simulink model "INS"  (R2021a)
settings: configuration reference "ins_config" (kept outside this file)
undefined symbols (not defined in the file): DiscIntNeverNeededParam, INS_CONST, INS_EXPORT, INS_EXPORT_VALUE, INS_PARAM
libraries: simulink x111, FMT_Model_Lib x36
(part 3 of 5)

== system INS/Data_Fusion/Rotation_Filter/RF_Data_PreProcess/Attitude_Reset/Reset Heading ==
  note: When GPS is valid at first time, the mag data will be compensated with WMM data,
      | so we need reset attitude.
  GPS_valid : Inport
  Add : Sum  AccumDataTypeStr=uint32
  Data Type Conversion : DataTypeConversion  OutDataTypeStr=uint32
  Delay : Delay  DelayLength=1
  Detect Rise Positive1 : simulink/Logic and Bit Operations/Detect Rise Positive  vinit=0  OutDataTypeStr=boolean
  Saturation : Saturate  UpperLimit=1  LowerLimit=0
  reset : Outport  VectorParamsAs1DForOutWhenUnconnected=off
  wires:
  Delay/1 -> Add/2
  Data Type Conversion/1 -> Add/1
  GPS_valid/1 -> Data Type Conversion/1
  Detect Rise Positive1/1 -> reset/1
  Add/1 -> Saturation/1
  Saturation/1 -> Detect Rise Positive1/1, Delay/1

== system INS/Data_Fusion/Rotation_Filter/RF_Data_PreProcess/Attitude_Reset/sample_valid ==
  valid : Inport
  Add : Sum  AccumDataTypeStr=uint32
  Data Type Conversion : DataTypeConversion  OutDataTypeStr=uint32
  Delay : Delay  DelayLength=1
  Saturation : Saturate  UpperLimit=10000  LowerLimit=0
  valid_samples : simulink/Logic and Bit Operations/Compare To Constant  relop=>  const=50  OutDataTypeStr=boolean
  sample_valid : Outport  VectorParamsAs1DForOutWhenUnconnected=off
  wires:
  Add/1 -> Saturation/1
  valid_samples/1 -> sample_valid/1
  Delay/1 -> Add/2
  valid/1 -> Data Type Conversion/1
  Data Type Conversion/1 -> Add/1
  Saturation/1 -> valid_samples/1, Delay/1

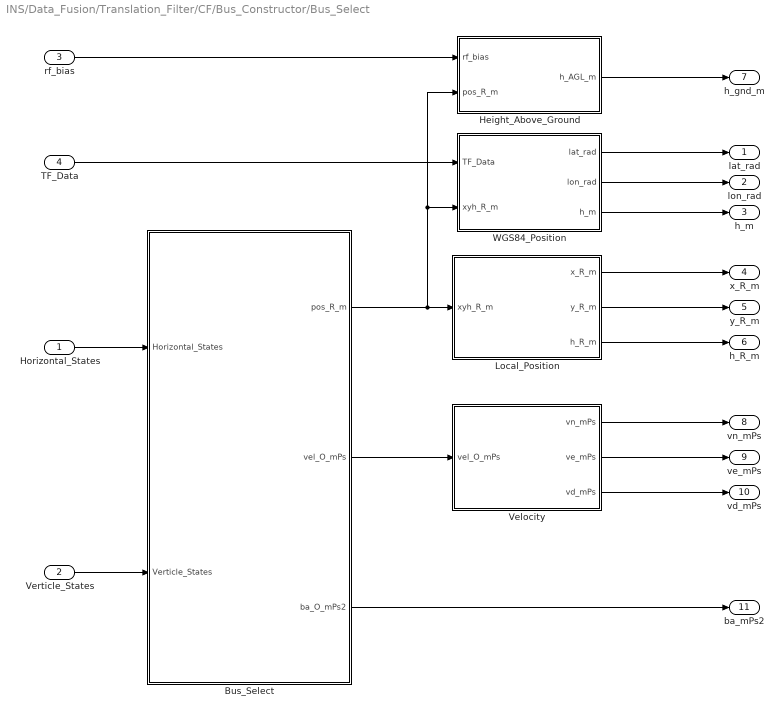
== system INS/Data_Fusion/Translation_Filter/CF/Bus_Constructor/Bus_Select ==
  Horizontal_States : Inport
  Verticle_States : Inport  Port=2
  rf_bias : Inport  Port=3
  TF_Data : Inport  Port=4
  Bus_Select : Subsystem
  Height_Above_Ground : Subsystem
  Local_Position : Subsystem
  Velocity : Subsystem
  WGS84_Position : Subsystem
  lat_rad : Outport  VectorParamsAs1DForOutWhenUnconnected=off
  lon_rad : Outport  Port=2  VectorParamsAs1DForOutWhenUnconnected=off
  h_m : Outport  Port=3  VectorParamsAs1DForOutWhenUnconnected=off
  x_R_m : Outport  Port=4  VectorParamsAs1DForOutWhenUnconnected=off
  y_R_m : Outport  Port=5  VectorParamsAs1DForOutWhenUnconnected=off
  h_R_m : Outport  Port=6  VectorParamsAs1DForOutWhenUnconnected=off
  h_gnd_m : Outport  Port=7  VectorParamsAs1DForOutWhenUnconnected=off
  vn_mPs : Outport  Port=8  VectorParamsAs1DForOutWhenUnconnected=off
  ve_mPs : Outport  Port=9  VectorParamsAs1DForOutWhenUnconnected=off
  vd_mPs : Outport  Port=10  VectorParamsAs1DForOutWhenUnconnected=off
  ba_mPs2 : Outport  Port=11  VectorParamsAs1DForOutWhenUnconnected=off
  wires:
  WGS84_Position/1(lat_rad) -> lat_rad/1
  TF_Data/1 -> WGS84_Position/1(TF_Data)
  WGS84_Position/2(lon_rad) -> lon_rad/1
  WGS84_Position/3(h_m) -> h_m/1
  Local_Position/1(x_R_m) -> x_R_m/1
  Local_Position/2(y_R_m) -> y_R_m/1
  Local_Position/3(h_R_m) -> h_R_m/1
  Bus_Select/1(pos_R_m) -> Local_Position/1(xyh_R_m), Height_Above_Ground/2(pos_R_m), WGS84_Position/2(xyh_R_m)
  Horizontal_States/1 -> Bus_Select/1(Horizontal_States)
  Verticle_States/1 -> Bus_Select/2(Verticle_States)
  Bus_Select/3(ba_O_mPs2) -> ba_mPs2/1
  Height_Above_Ground/1(h_AGL_m) -> h_gnd_m/1
  Bus_Select/2(vel_O_mPs) -> Velocity/1(vel_O_mPs)
  Velocity/1(vn_mPs) -> vn_mPs/1
  Velocity/2(ve_mPs) -> ve_mPs/1
  Velocity/3(vd_mPs) -> vd_mPs/1
  rf_bias/1 -> Height_Above_Ground/1(rf_bias)

== system INS/Data_Fusion/Translation_Filter/CF/Horizontal_Filter/Correct ==
  X_Predict : Inport
  TF_Data : Inport  Port=2
  GPS Correct : Subsystem
  OptFlow Correct : Subsystem
  X_Next : Outport  VectorParamsAs1DForOutWhenUnconnected=off
  wires:
  GPS Correct/1(X_Next) -> X_Next/1
  X_Predict/1 -> OptFlow Correct/1(X_Predict)
  OptFlow Correct/1(X_Next) -> GPS Correct/1(X_Predict)
  TF_Data/1 -> GPS Correct/2(TF_Data), OptFlow Correct/2(TF_Data)

== system INS/Data_Fusion/Translation_Filter/CF/Horizontal_Filter/Predict ==
  X_Prio : Inport
  Rotation_Data : Inport  Port=2
  TF_Data : Inport  Port=3
  Propagate : Subsystem
  Update : Subsystem
  X_Predict : Outport  VectorParamsAs1DForOutWhenUnconnected=off
  wires:
  X_Prio/1 -> Propagate/1(X_prio)
  TF_Data/1 -> Propagate/2(TF_Data)
  Propagate/1(X) -> Update/1(X_Prio)
  Rotation_Data/1 -> Update/2(Rotation_Data)
  Update/1(X_Predict) -> X_Predict/1

== system INS/Data_Fusion/Translation_Filter/CF/Verticle_Filter/Correct ==
  X_Predict : Inport
  TF_Data : Inport  Port=2
  Baro_Correct : Subsystem
  GPS_Correct : Subsystem
  Rf_Correct : Subsystem
  X_Next : Outport  VectorParamsAs1DForOutWhenUnconnected=off
  rf_bias : Outport  Port=2  VectorParamsAs1DForOutWhenUnconnected=off
  wires:
  TF_Data/1 -> Rf_Correct/2(TF_Data), GPS_Correct/2(TF_Data), Baro_Correct/2(TF_Data)
  X_Predict/1 -> Baro_Correct/1(X_Predict)
  Baro_Correct/1(X_Next) -> GPS_Correct/1(X_Predict)
  GPS_Correct/1(X_Next) -> Rf_Correct/1(X_Predict)
  Rf_Correct/1(X_Next) -> X_Next/1
  Rf_Correct/2(rf_bias) -> rf_bias/1

== system INS/Data_Fusion/Translation_Filter/CF/Verticle_Filter/Predict ==
  X_Prio : Inport
  Rotation_Data : Inport  Port=2
  TF_Data : Inport  Port=3
  Propagate : Subsystem
  Update : Subsystem
  X_Predict : Outport  VectorParamsAs1DForOutWhenUnconnected=off
  wires:
  X_Prio/1 -> Propagate/1(X_Prio)
  TF_Data/1 -> Propagate/2(TF_Data)
  Propagate/1(X) -> Update/1(X_Prio)
  Rotation_Data/1 -> Update/2(Rotation_Data)
  Update/1(X_Predict) -> X_Predict/1

== system INS/Data_Fusion/Translation_Filter/TF_Data_PreProcess/Sensor_Process/Sensor_Select ==
  Sensor_Status : Inport
  Bus Creator : BusCreator  Inputs=2
  Horizontal_Sensor_Select : Subsystem
  Vertical_Sensor_Select : Subsystem
  Sensor_Select : Outport  VectorParamsAs1DForOutWhenUnconnected=off
  wires:
  Sensor_Status/1 -> Vertical_Sensor_Select/1(Sensor_Status), Horizontal_Sensor_Select/1(Sensor_Status)
  Bus Creator/1 -> Sensor_Select/1
  Horizontal_Sensor_Select/1(horizon_select) -> Bus Creator/1  "horizon_select"
  Vertical_Sensor_Select/1(vert_select) -> Bus Creator/2  "vert_select"

== system INS/Data_Fusion/Translation_Filter/TF_Data_PreProcess/Sensor_Process/TF_Sensor_Measures ==
  Sensor_Data : Inport
  Rotation_Data : Inport  Port=2
  Barometer_Meas : Subsystem
  Bus Creator : BusCreator  Inputs=4
  GPS_Meas : Subsystem
  OpticalFlow_Meas : Subsystem
  Rangefinder_Meas : Subsystem
  Sensor_Meas : Outport  VectorParamsAs1DForOutWhenUnconnected=off
  wires:
  Bus Creator/1 -> Sensor_Meas/1
  Sensor_Data/1 -> OpticalFlow_Meas/1(Sensor_Data), Rangefinder_Meas/1(Sensor_Data), Barometer_Meas/1(Sensor_Data), GPS_Meas/1(Sensor_Data)
  GPS_Meas/1(GPS_Meas) -> Bus Creator/1  "GPS_Meas"
  Barometer_Meas/1(Baro_Meas) -> Bus Creator/2  "Baro_Meas"
  Rangefinder_Meas/1(Rf_Meas) -> Bus Creator/3  "Rf_Meas"
  OpticalFlow_Meas/1(OptFlow_Meas) -> Bus Creator/4  "OptFlow_Meas"
  Rotation_Data/1 -> OpticalFlow_Meas/2(Rotation_Data)

== system INS/Data_Fusion/Translation_Filter/TF_Data_PreProcess/Sensor_Process/TF_Sensor_Status ==
  Sensor_Data : Inport
  Barometer_Status : Subsystem
  Bus Creator : BusCreator  Inputs=4
  GPS_Status : Subsystem
  OpticalFlow_Status : Subsystem
  Rangefinder_Status : Subsystem
  Sensor_Status : Outport  VectorParamsAs1DForOutWhenUnconnected=off
  wires:
  Bus Creator/1 -> Sensor_Status/1
  Sensor_Data/1 -> OpticalFlow_Status/1(Sensor_Data), Rangefinder_Status/1(Sensor_Data), Barometer_Status/1(Sensor_Data), GPS_Status/1(Sensor_Data)
  GPS_Status/1(GPS_Status) -> Bus Creator/1  "GPS_Status"
  Barometer_Status/1(Baro_Status) -> Bus Creator/2  "Baro_Status"
  Rangefinder_Status/1(Rf_Status) -> Bus Creator/3  "Rf_Status"
  OpticalFlow_Status/1(OptFlow_Status) -> Bus Creator/4  "OptFlow_Status"

== system INS/Data_Fusion/Translation_Filter/TF_Data_PreProcess/Transfer_Filter_Control/Filter_Reset ==
  note: Height_Reset
  note: Position_Reset
  Sensor_Valid : Inport
  Bus Selector : BusSelector  OutputSignals=xy_R_valid
  Bus Selector1 : BusSelector  OutputSignals=h_R_valid
  Detect Rise Positive : simulink/Logic and Bit Operations/Detect Rise Positive  vinit=0  OutDataTypeStr=boolean
  Detect Rise Positive1 : simulink/Logic and Bit Operations/Detect Rise Positive  vinit=0  OutDataTypeStr=boolean
  pos_reset : Outport  VectorParamsAs1DForOutWhenUnconnected=off
  height_reset : Outport  Port=2  VectorParamsAs1DForOutWhenUnconnected=off
  wires:
  Detect Rise Positive/1 -> pos_reset/1
  Detect Rise Positive1/1 -> height_reset/1
  Bus Selector/1 -> Detect Rise Positive/1  "<xy_R_valid>"
  Bus Selector1/1 -> Detect Rise Positive1/1  "<h_R_valid>"
  Sensor_Valid/1 -> Bus Selector1/1, Bus Selector/1

== system INS/Data_Fusion/Translation_Filter/TF_Data_PreProcess/Transfer_Filter_Control/Sensor_Valid ==
  Sensor_Enable : Inport
  Bus Creator : BusCreator  Inputs=5
  Horizon_Sensor_Valid : Subsystem
  Vertical_Sensor_Valid : Subsystem
  Sensor_Valid : Outport  VectorParamsAs1DForOutWhenUnconnected=off
  wires:
  Horizon_Sensor_Valid/1(lon_lat_valid) -> Bus Creator/1  "lon_lat_valid"
  Horizon_Sensor_Valid/2(xy_R_valid) -> Bus Creator/2  "xy_R_valid"
  Vertical_Sensor_Valid/1(altitude_valid) -> Bus Creator/3  "altitude_valid"
  Vertical_Sensor_Valid/2(h_R_valid) -> Bus Creator/4  "h_R_valid"
  Bus Creator/1 -> Sensor_Valid/1
  Sensor_Enable/1 -> Horizon_Sensor_Valid/1(Sensor_Enable), Vertical_Sensor_Valid/1(Sensor_Enable)
  Vertical_Sensor_Valid/3(h_AGL_valid) -> Bus Creator/5  "h_AGL_valid"

== system INS/Data_Fusion/Translation_Filter/TF_Data_PreProcess/Transfer_Filter_Control/WGS84_Reference ==
  Sensor_Valid : Inport
  Translation_Data : Inport  Port=2
  Sensor_Meas : Inport  Port=3
  Bus_Constructor : Subsystem
  Bus_Select : Subsystem
  Height_Ref : Subsystem
  Position_Ref : Subsystem
  WGS84_Ref : Outport  VectorParamsAs1DForOutWhenUnconnected=off
  wires:
  Bus_Select/2(WGS84_position) -> Position_Ref/4(WGS84_position), Height_Ref/4(WGS84_position)
  Translation_Data/1 -> Height_Ref/1(Translation_Data), Position_Ref/1(Translation_Data)
  Sensor_Valid/1 -> Height_Ref/2(Sensor_Valid), Position_Ref/2(Sensor_Valid)
  Bus_Select/1(WGS84_derivatives) -> Height_Ref/3(WGS84_derivatives), Position_Ref/3(WGS84_derivatives)
  Position_Ref/1(WGS84_pos_ref) -> Bus_Constructor/1(WGS84_pos_ref)
  Position_Ref/2(WGS84_dpos_ref) -> Bus_Constructor/2(WGS84_dpos_ref)
  Height_Ref/1(WGS84_hgt_ref) -> Bus_Constructor/3(WGS84_hgt_ref)
  Height_Ref/2(WGS84_dhgt_ref) -> Bus_Constructor/4(WGS84_dhgt_ref)
  Bus_Constructor/1(WGS84_Ref) -> WGS84_Ref/1
  Sensor_Meas/1 -> Bus_Select/1(Sensor_Meas)

== system INS/Sensor_PreProcess/GPS_PreProcess/Status_Quality/GPS_Status/Ready ==
  valid : Inport
  Saturation : Saturate  UpperLimit=1e4  LowerLimit=0
  Sum : Sum  Inputs=|++  OutDataTypeStr=int32
  Unit Delay : UnitDelay  SampleTime=-1  HasFrameUpgradeWarning=on
  valid_samples : simulink/Logic and Bit Operations/Compare To Constant  relop=>=  const=1000  OutDataTypeStr=boolean
  ready : Outport  VectorParamsAs1DForOutWhenUnconnected=off
  wires:
  valid_samples/1 -> ready/1
  Sum/1 -> Saturation/1
  Unit Delay/1 -> valid_samples/1, Sum/2
  Saturation/1 -> Unit Delay/1
  valid/1 -> Sum/1

== system INS/Sensor_PreProcess/MAG_PreProcess/Mag_Data_Process/Mag_Quality_Estimate/Mag_Quality ==
  nominal_inc_deg : Inport
  mag_normalized_O : Inport  Port=2
  Inclination_Quality_Estimate : Subsystem
  Intensity_Quality_Estimate : Subsystem
  MinMax : MinMax  Inputs=2
  Second Order LPF : FMT_Model_Lib/Filter/Second Order LPF  fc=5  zeta=0.707
      settings: SourceProductName=FMT Toolbox
  mag_quality : Outport  VectorParamsAs1DForOutWhenUnconnected=off
  wires:
  Intensity_Quality_Estimate/1(intensity_quality) -> MinMax/2  "mag_int_quality"
  nominal_inc_deg/1 -> Inclination_Quality_Estimate/1(nominal_inc_deg)
  Inclination_Quality_Estimate/1(inclination_quality) -> MinMax/1  "mag_inc_quality"
  mag_normalized_O/1 -> Inclination_Quality_Estimate/2(mag_normalized_O), Intensity_Quality_Estimate/1(mag_normalized_O)
  MinMax/1 -> Second Order LPF/1
  Second Order LPF/1 -> mag_quality/1

== system INS/Sensor_PreProcess/MAG_PreProcess/Mag_Data_Process/WMM_Compensation/safe_divide ==
  u1 : Inport
  u2 : Inport  Port=2
  Constant1 : Constant  VectorParams1D=off  OutDataTypeStr=single
  Divide1 : Product  Inputs=*/
  MinMax : MinMax  Function=max  Inputs=2
  y : Outport  VectorParamsAs1DForOutWhenUnconnected=off
  wires:
  MinMax/1 -> Divide1/2
  Constant1/1 -> MinMax/1
  Divide1/1 -> y/1
  u2/1 -> MinMax/2
  u1/1 -> Divide1/1

== system INS/Data_Fusion/Rotation_Filter/AHRS/Correct/Attitude_Correction/Attitude_Correct ==
  Rotation_Data : Inport
  Sensor_Data : Inport  Port=2
  Acc_Correct : Subsystem
  Acc_Estimator : Subsystem
  att_corr_O : Outport  VectorParamsAs1DForOutWhenUnconnected=off
  wires:
  Acc_Estimator/3(acc_est_O_mPs2) -> Acc_Correct/3(acc_est_O_mPs2)  "acc_est_O_mPs2"
  Sensor_Data/1 -> Acc_Estimator/1(Sensor_Data)
  Rotation_Data/1 -> Acc_Estimator/2(Rotation_Data)
  Acc_Correct/1(att_correct) -> att_corr_O/1
  Acc_Estimator/1(acc_meas_valid) -> Acc_Correct/1(acc_meas_valid)  "acc_meas_valid"
  Acc_Estimator/2(acc_meas_O_mPs2) -> Acc_Correct/2(acc_meas_O_mPs2)  "acc_meas_O_mPs2"

== system INS/Data_Fusion/Rotation_Filter/AHRS/Correct/Attitude_Correction/Mag_Correct ==
  Rotation_Data : Inport
  Sensor_Data : Inport  Port=2
  standstill : Inport  Port=3
  Bus Selector1 : BusSelector  OutputSignals=Mag_Data.mag_norm_B,Mag_Data.mag_quality
  Bus Selector4 : BusSelector  OutputSignals=M_OB
  Constant : Constant  Value=INS_PARAM.MAG_AIR_EN
  Logical Operator : Logic  AllPortsSameDT=off  OutDataTypeStr=boolean
  Logical Operator1 : Logic  Operator=OR  AllPortsSameDT=off  OutDataTypeStr=boolean
  MX Product3 : Product  Inputs=3  RndMeth=Simplest
  MX Product4 : Product  Multiplication=Matrix(*)  RndMeth=Simplest
  Relay1 : Relay  OnSwitchValue=0.3  OffSwitchValue=0.2
  Selector4 : Selector  NumberOfDimensions=2  InputPortWidth=3  IndexOptions=Index vector (dialog),Index vector (dialog)  Indices=[2],[1 2 3]  OutputSizes=1,1
  Subsystem : Subsystem  Commented=on
  Z axis : Constant  Value=[0 0 1]  OutDataTypeStr=single
  mag_correct_gain : Gain  Gain=-INS_PARAM.MAG_GAIN  OutDataTypeStr=Inherit: Same as input
  mag_corr_O : Outport  VectorParamsAs1DForOutWhenUnconnected=off
  wires:
  Bus Selector4/1 -> Subsystem/1(M_OB), Selector4/1  "<M_OB>"
  Rotation_Data/1 -> Subsystem/3(Rotation_Data), Bus Selector4/1
  Bus Selector1/2 -> Relay1/1  "<mag_quality>"
  Sensor_Data/1 -> Bus Selector1/1
  mag_correct_gain/1 -> MX Product3/2
  MX Product4/1 -> mag_correct_gain/1  "my_O"
  Selector4/1 -> MX Product4/1
  Relay1/1 -> Logical Operator/1  "mag_enable"
  Logical Operator/1 -> MX Product3/3
  Logical Operator1/1 -> Logical Operator/2
  Constant/1 -> Logical Operator1/1
  standstill/1 -> Logical Operator1/2
  MX Product3/1 -> mag_corr_O/1
  Bus Selector1/1 -> Subsystem/2(mag_B), MX Product4/2  "<mag_norm_B>"
  Z axis/1 -> MX Product3/1

== system INS/Data_Fusion/Translation_Filter/CF/Bus_Constructor/Bus_Select/Bus_Select ==
  Horizontal_States : Inport
  Verticle_States : Inport  Port=2
  Mux : Mux  Inputs=2
  Mux1 : Mux  Inputs=2
  Mux2 : Mux  Inputs=2
  Selector : Selector  InputPortWidth=6  IndexOptions=Index vector (dialog)  Indices=[1 2]  OutputSizes=1
  Selector1 : Selector  InputPortWidth=3  IndexOptions=Index vector (dialog)  Indices=[1]  OutputSizes=1
  Selector2 : Selector  InputPortWidth=6  IndexOptions=Index vector (dialog)  Indices=[3 4]  OutputSizes=1
  Selector3 : Selector  InputPortWidth=3  IndexOptions=Index vector (dialog)  Indices=[2]  OutputSizes=1
  Selector4 : Selector  InputPortWidth=6  IndexOptions=Index vector (dialog)  Indices=[5 6]  OutputSizes=1
  Selector5 : Selector  InputPortWidth=3  IndexOptions=Index vector (dialog)  Indices=[3]  OutputSizes=1
  pos_R_m : Outport  VectorParamsAs1DForOutWhenUnconnected=off
  vel_O_mPs : Outport  Port=2  VectorParamsAs1DForOutWhenUnconnected=off
  ba_O_mPs2 : Outport  Port=3  VectorParamsAs1DForOutWhenUnconnected=off
  wires:
  Selector5/1 -> Mux2/2
  Horizontal_States/1 -> Selector4/1, Selector2/1, Selector/1
  Selector4/1 -> Mux2/1
  Selector2/1 -> Mux1/1
  Selector1/1 -> Mux/2
  Selector/1 -> Mux/1
  Selector3/1 -> Mux1/2
  Mux1/1 -> vel_O_mPs/1
  Verticle_States/1 -> Selector5/1, Selector3/1, Selector1/1
  Mux/1 -> pos_R_m/1
  Mux2/1 -> ba_O_mPs2/1

== system INS/Data_Fusion/Translation_Filter/CF/Bus_Constructor/Bus_Select/Height_Above_Ground ==
  rf_bias : Inport
  pos_R_m : Inport  Port=2
  Selector : Selector  InputPortWidth=3  IndexOptions=Index vector (dialog)  Indices=3  OutputSizes=1
  Sum : Sum  Inputs=|-+
  h_AGL_m : Outport  VectorParamsAs1DForOutWhenUnconnected=off
  wires:
  rf_bias/1 -> Sum/1
  pos_R_m/1 -> Selector/1
  Sum/1 -> h_AGL_m/1
  Selector/1 -> Sum/2

== system INS/Data_Fusion/Translation_Filter/CF/Bus_Constructor/Bus_Select/Local_Position ==
  xyh_R_m : Inport
  Demux : Demux  Outputs=3
  x_R_m : Outport  VectorParamsAs1DForOutWhenUnconnected=off
  y_R_m : Outport  Port=2  VectorParamsAs1DForOutWhenUnconnected=off
  h_R_m : Outport  Port=3  VectorParamsAs1DForOutWhenUnconnected=off
  wires:
  Demux/2 -> y_R_m/1
  Demux/1 -> x_R_m/1
  Demux/3 -> h_R_m/1
  xyh_R_m/1 -> Demux/1

== system INS/Data_Fusion/Translation_Filter/CF/Bus_Constructor/Bus_Select/Velocity ==
  vel_O_mPs : Inport
  Demux : Demux  Outputs=3
  vn_mPs : Outport  VectorParamsAs1DForOutWhenUnconnected=off
  ve_mPs : Outport  Port=2  VectorParamsAs1DForOutWhenUnconnected=off
  vd_mPs : Outport  Port=3  VectorParamsAs1DForOutWhenUnconnected=off
  wires:
  Demux/3 -> vd_mPs/1
  Demux/1 -> vn_mPs/1
  Demux/2 -> ve_mPs/1
  vel_O_mPs/1 -> Demux/1

== system INS/Data_Fusion/Translation_Filter/CF/Bus_Constructor/Bus_Select/WGS84_Position ==
  TF_Data : Inport
  xyh_R_m : Inport  Port=2
  Bus Selector2 : BusSelector  OutputSignals=Sensor_Status.GPS_Status.gps_vaid
  Data Type Conversion2 : DataTypeConversion  OutDataTypeStr=double
  Demux2 : Demux  Outputs=3
  Multiply : Product
  WGS84_Position : Subsystem
  lat_rad : Outport  VectorParamsAs1DForOutWhenUnconnected=off
  lon_rad : Outport  Port=2  VectorParamsAs1DForOutWhenUnconnected=off
  h_m : Outport  Port=3  VectorParamsAs1DForOutWhenUnconnected=off
  wires:
  WGS84_Position/1(WGS84_pos) -> Multiply/2
  TF_Data/1 -> Bus Selector2/1, WGS84_Position/2(TF_Data)
  Bus Selector2/1 -> Data Type Conversion2/1  "<gps_vaid>"
  Data Type Conversion2/1 -> Multiply/1
  Multiply/1 -> Demux2/1
  xyh_R_m/1 -> WGS84_Position/1(xyh_R_m)
  Demux2/1 -> lat_rad/1  "lat_rad"
  Demux2/2 -> lon_rad/1  "lon_rad"
  Demux2/3 -> h_m/1  "h_m"

== system INS/Data_Fusion/Translation_Filter/CF/Horizontal_Filter/Correct/GPS Correct ==
  X_Predict : Inport
  TF_Data : Inport  Port=2
  Bus Selector : BusSelector  OutputSignals=Sensor_Enable.horizon_select.gps_enable
  GPS_Correct : Subsystem
  Switch : Switch  Criteria=u2 > Threshold
  X_Next : Outport  VectorParamsAs1DForOutWhenUnconnected=off
  wires:
  GPS_Correct/1(X_Next) -> Switch/1
  Switch/1 -> X_Next/1
  X_Predict/1 -> GPS_Correct/2(X_Predict), Switch/3
  Bus Selector/1 -> GPS_Correct/Enable, Switch/2  "<gps_enable>"
  TF_Data/1 -> GPS_Correct/1(TF_Data), Bus Selector/1

== system INS/Data_Fusion/Translation_Filter/CF/Horizontal_Filter/Correct/OptFlow Correct ==
  X_Predict : Inport
  TF_Data : Inport  Port=2
  Bus Selector : BusSelector  OutputSignals=Sensor_Enable.horizon_select.optflow_enable
  OptFlow_Correct : Subsystem
  Switch : Switch  Criteria=u2 > Threshold
  X_Next : Outport  VectorParamsAs1DForOutWhenUnconnected=off
  wires:
  OptFlow_Correct/1(X_Next) -> Switch/1
  Switch/1 -> X_Next/1
  X_Predict/1 -> OptFlow_Correct/2(X_Predict), Switch/3
  Bus Selector/1 -> OptFlow_Correct/Enable, Switch/2  "<optflow_enable>"
  TF_Data/1 -> OptFlow_Correct/1(TF_Data), Bus Selector/1

== system INS/Data_Fusion/Translation_Filter/CF/Horizontal_Filter/Predict/Propagate ==
  X_prio : Inport
  TF_Data : Inport  Port=2
  Bus Selector : BusSelector  OutputSignals=TF_Control.pos_reset
  Delay : Delay  DelayLength=1
  States_Init : Subsystem
  Switch : Switch  Criteria=u2 > Threshold
  X : Outport  VectorParamsAs1DForOutWhenUnconnected=off
  wires:
  Delay/1 -> Switch/3
  States_Init/1(X_0) -> Switch/1
  Switch/1 -> X/1
  Bus Selector/1 -> Switch/2  "<pos_reset>"
  TF_Data/1 -> Bus Selector/1, States_Init/1(TF_Data)
  X_prio/1 -> Delay/1

== system INS/Data_Fusion/Translation_Filter/CF/Horizontal_Filter/Predict/Update ==
  X_Prio : Inport
  Rotation_Data : Inport  Port=2
  Add : Sum  Inputs=-+
  Bus Selector2 : BusSelector  OutputSignals=M_OB,acc_B_mPs2
  Constant : Constant  Value=[0;0]  OutDataTypeStr=single
  Gain : Gain  Gain=INS_CONST.dt  OutDataTypeStr=Inherit: Same as input
  Multiply : Product  Multiplication=Matrix(*)
  Mux : Mux  Inputs=3
  Reshape : Reshape  OutputDimensionality=Customize  OutputDimensions=[6,1]
  Selector : Selector  InputPortWidth=3  IndexOptions=Index vector (dialog)  Indices=[1 2]  OutputSizes=1
  Selector1 : Selector  InputPortWidth=6  IndexOptions=Index vector (dialog)  Indices=[3 4]  OutputSizes=1
  Selector2 : Selector  InputPortWidth=6  IndexOptions=Index vector (dialog)  Indices=[5 6]  OutputSizes=1
  Sum : Sum  Inputs=++|
  X_Predict : Outport  VectorParamsAs1DForOutWhenUnconnected=off
  wires:
  Rotation_Data/1 -> Bus Selector2/1
  Bus Selector2/1 -> Multiply/1  "<M_OB>"
  Multiply/1 -> Selector/1  "acc_O"
  Bus Selector2/2 -> Multiply/2  "<acc_B_mPs2>"
  X_Prio/1 -> Selector1/1, Sum/1, Selector2/1
  Selector/1 -> Add/2
  Selector1/1 -> Mux/1
  Constant/1 -> Mux/3
  Mux/1 -> Reshape/1
  Reshape/1 -> Gain/1
  Sum/1 -> X_Predict/1
  Gain/1 -> Sum/2
  Add/1 -> Mux/2
  Selector2/1 -> Add/1

== system INS/Data_Fusion/Translation_Filter/CF/Verticle_Filter/Correct/Baro_Correct ==
  X_Predict : Inport
  TF_Data : Inport  Port=2
  Baro_Correct : Subsystem
  Bus Selector : BusSelector  OutputSignals=Sensor_Enable.vert_select.baro_enable
  Switch : Switch  Criteria=u2 > Threshold
  X_Next : Outport  VectorParamsAs1DForOutWhenUnconnected=off
  wires:
  Switch/1 -> X_Next/1
  Bus Selector/1 -> Baro_Correct/Enable, Switch/2  "<baro_enable>"
  TF_Data/1 -> Baro_Correct/1(TF_Data), Bus Selector/1
  Baro_Correct/1(X_Next) -> Switch/1
  X_Predict/1 -> Baro_Correct/2(X_Predict), Switch/3

== system INS/Data_Fusion/Translation_Filter/CF/Verticle_Filter/Correct/GPS_Correct ==
  X_Predict : Inport
  TF_Data : Inport  Port=2
  Bus Selector : BusSelector  OutputSignals=Sensor_Enable.vert_select.gps_enable
  GPS_Correct : Subsystem
  Switch : Switch  Criteria=u2 > Threshold
  X_Next : Outport  VectorParamsAs1DForOutWhenUnconnected=off
  wires:
  Switch/1 -> X_Next/1
  Bus Selector/1 -> GPS_Correct/Enable, Switch/2  "<gps_enable>"
  TF_Data/1 -> GPS_Correct/1(TF_Data), Bus Selector/1
  GPS_Correct/1(X_Next) -> Switch/1
  X_Predict/1 -> GPS_Correct/2(X_Predict), Switch/3

== system INS/Data_Fusion/Translation_Filter/CF/Verticle_Filter/Correct/Rf_Correct ==
  X_Predict : Inport
  TF_Data : Inport  Port=2
  Bus Selector : BusSelector  OutputSignals=Sensor_Enable.vert_select.rf_enable
  Rangefinder_Correct : Subsystem
  Switch : Switch  Criteria=u2 > Threshold
  X_Next : Outport  VectorParamsAs1DForOutWhenUnconnected=off
  rf_bias : Outport  Port=2  VectorParamsAs1DForOutWhenUnconnected=off
  wires:
  Switch/1 -> X_Next/1
  Bus Selector/1 -> Rangefinder_Correct/Enable, Switch/2  "<rf_enable>"
  TF_Data/1 -> Rangefinder_Correct/1(TF_Data), Bus Selector/1
  Rangefinder_Correct/1(X_Next) -> Switch/1
  X_Predict/1 -> Rangefinder_Correct/2(X_Predict), Switch/3
  Rangefinder_Correct/2(rf_bias) -> rf_bias/1

== system INS/Data_Fusion/Translation_Filter/CF/Verticle_Filter/Predict/Propagate ==
  X_Prio : Inport
  TF_Data : Inport  Port=2
  Bus Selector : BusSelector  OutputSignals=TF_Control.height_reset
  Delay : Delay  DelayLength=1
  States_Init : Subsystem
  Switch : Switch  Criteria=u2 > Threshold
  X : Outport  VectorParamsAs1DForOutWhenUnconnected=off
  wires:
  X_Prio/1 -> Delay/1
  TF_Data/1 -> States_Init/1(TF_Data), Bus Selector/1
  Bus Selector/1 -> Switch/2  "<height_reset>"
  Switch/1 -> X/1
  States_Init/1(X_0) -> Switch/1
  Delay/1 -> Switch/3

== system INS/Data_Fusion/Translation_Filter/CF/Verticle_Filter/Predict/Update ==
  X_Prio : Inport
  Rotation_Data : Inport  Port=2
  Add : Sum  Inputs=-++
  Bus Selector2 : BusSelector  OutputSignals=M_OB,acc_B_mPs2
  Constant : Constant  Value=0  OutDataTypeStr=single
  Constant1 : Constant  Value=INS_CONST.g  OutDataTypeStr=single
  Gain : Gain  Gain=INS_CONST.dt  OutDataTypeStr=Inherit: Same as input
  Gain1 : Gain  Gain=-1  OutDataTypeStr=Inherit: Same as input
  Multiply : Product  Multiplication=Matrix(*)
  Mux : Mux  Inputs=3
  Reshape : Reshape  OutputDimensionality=Customize  OutputDimensions=[3,1]
  Selector : Selector  InputPortWidth=3  IndexOptions=Index vector (dialog)  Indices=[3]  OutputSizes=1
  Selector1 : Selector  InputPortWidth=3  IndexOptions=Index vector (dialog)  Indices=[2]  OutputSizes=1
  Selector2 : Selector  InputPortWidth=3  IndexOptions=Index vector (dialog)  Indices=[3]  OutputSizes=1
  Sum : Sum  Inputs=++|
  X_Predict : Outport  VectorParamsAs1DForOutWhenUnconnected=off
  wires:
  Rotation_Data/1 -> Bus Selector2/1
  Bus Selector2/1 -> Multiply/1  "<M_OB>"
  Multiply/1 -> Selector/1  "acc_O"
  Bus Selector2/2 -> Multiply/2  "<acc_B_mPs2>"
  X_Prio/1 -> Selector2/1, Sum/1, Selector1/1
  Selector1/1 -> Gain1/1
  Constant/1 -> Mux/3
  Mux/1 -> Reshape/1
  Reshape/1 -> Gain/1
  Sum/1 -> X_Predict/1
  Add/1 -> Mux/2
  Constant1/1 -> Add/3
  Selector2/1 -> Add/1  "bias_az"
  Gain1/1 -> Mux/1
  Gain/1 -> Sum/2
  Selector/1 -> Add/2

== system INS/Data_Fusion/Translation_Filter/TF_Data_PreProcess/Sensor_Process/Sensor_Select/Horizontal_Sensor_Select ==
  Sensor_Status : Inport
  Bus Creator : BusCreator  Inputs=2
  Bus Selector : BusSelector  OutputSignals=GPS_Status.gps_vaid,GPS_Status.spd_valid,GPS_Status.pos_valid
  Bus Selector1 : BusSelector  OutputSignals=OptFlow_Status.optflow_valid
  Compare To Zero2 : simulink/Logic and Bit Operations/Compare To Zero  relop=>  OutDataTypeStr=boolean
  Compare To Zero3 : simulink/Logic and Bit Operations/Compare To Zero  relop=>  OutDataTypeStr=boolean
  Compare To Zero4 : simulink/Logic and Bit Operations/Compare To Zero  relop=>  OutDataTypeStr=boolean
  Data Type Conversion1 : DataTypeConversion  OutDataTypeStr=int8
  Data Type Conversion2 : DataTypeConversion  OutDataTypeStr=int8
  Logical Operator : Logic  Inputs=3  AllPortsSameDT=off  OutDataTypeStr=boolean
  Saturation : Saturate  UpperLimit=1  LowerLimit=0
  Subtract1 : Sum  Inputs=-+
  horizon_select : Outport  VectorParamsAs1DForOutWhenUnconnected=off
  wires:
  Bus Selector/1 -> Logical Operator/1  "<gps_vaid>"
  Logical Operator/1 -> Data Type Conversion2/1
  Compare To Zero2/1 -> Bus Creator/1  "gps_enable"
  Sensor_Status/1 -> Bus Selector1/1, Bus Selector/1
  Bus Creator/1 -> horizon_select/1
  Bus Selector/2 -> Logical Operator/2  "<spd_valid>"
  Bus Selector/3 -> Logical Operator/3  "<pos_valid>"
  Subtract1/1 -> Saturation/1
  Data Type Conversion1/1 -> Subtract1/2
  Bus Selector1/1 -> Compare To Zero4/1  "<optflow_valid>"
  Compare To Zero4/1 -> Data Type Conversion1/1
  Saturation/1 -> Compare To Zero3/1
  Compare To Zero3/1 -> Bus Creator/2  "optflow_enable"
  Data Type Conversion2/1 -> Compare To Zero2/1, Subtract1/1

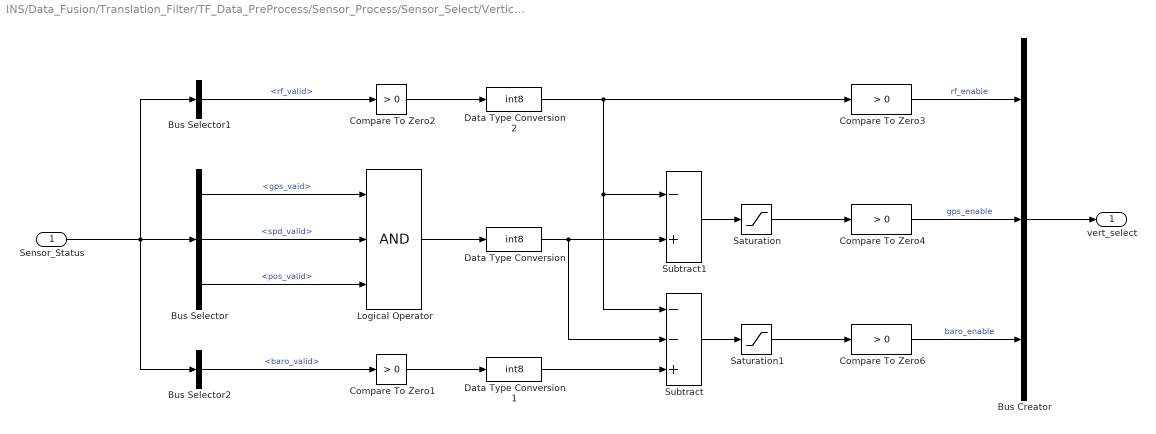
== system INS/Data_Fusion/Translation_Filter/TF_Data_PreProcess/Sensor_Process/Sensor_Select/Vertical_Sensor_Select ==
  Sensor_Status : Inport
  Bus Creator : BusCreator  Inputs=3
  Bus Selector : BusSelector  OutputSignals=GPS_Status.gps_vaid,GPS_Status.spd_valid,GPS_Status.pos_valid
  Bus Selector1 : BusSelector  OutputSignals=Rf_Status.rf_valid
  Bus Selector2 : BusSelector  OutputSignals=Baro_Status.baro_valid
  Compare To Zero{1..4,6} (5 alike) : simulink/Logic and Bit Operations/Compare To Zero  relop=>  OutDataTypeStr=boolean
  Data Type Conversion : DataTypeConversion  OutDataTypeStr=int8
  Data Type Conversion1 : DataTypeConversion  OutDataTypeStr=int8
  Data Type Conversion2 : DataTypeConversion  OutDataTypeStr=int8
  Logical Operator : Logic  Inputs=3  AllPortsSameDT=off  OutDataTypeStr=boolean
  Saturation : Saturate  UpperLimit=1  LowerLimit=0
  Saturation1 : Saturate  UpperLimit=1  LowerLimit=0
  Subtract : Sum  Inputs=--+
  Subtract1 : Sum  Inputs=-+
  vert_select : Outport  VectorParamsAs1DForOutWhenUnconnected=off
  wires:
  Logical Operator/1 -> Data Type Conversion/1
  Subtract1/1 -> Saturation/1
  Bus Selector/2 -> Logical Operator/2  "<spd_valid>"
  Bus Selector2/1 -> Compare To Zero1/1  "<baro_valid>"
  Compare To Zero1/1 -> Data Type Conversion1/1
  Subtract/1 -> Saturation1/1
  Saturation1/1 -> Compare To Zero6/1
  Data Type Conversion1/1 -> Subtract/3
  Bus Selector/1 -> Logical Operator/1  "<gps_vaid>"
  Bus Selector/3 -> Logical Operator/3  "<pos_valid>"
  Compare To Zero4/1 -> Bus Creator/2  "gps_enable"
  Compare To Zero6/1 -> Bus Creator/3  "baro_enable"
  Sensor_Status/1 -> Bus Selector1/1, Bus Selector/1, Bus Selector2/1
  Bus Creator/1 -> vert_select/1
  Bus Selector1/1 -> Compare To Zero2/1  "<rf_valid>"
  Compare To Zero2/1 -> Data Type Conversion2/1
  Data Type Conversion/1 -> Subtract/2, Subtract1/2
  Data Type Conversion2/1 -> Compare To Zero3/1, Subtract/1, Subtract1/1
  Saturation/1 -> Compare To Zero4/1
  Compare To Zero3/1 -> Bus Creator/1  "rf_enable"

== system INS/Data_Fusion/Translation_Filter/TF_Data_PreProcess/Sensor_Process/TF_Sensor_Measures/Barometer_Meas ==
  Sensor_Data : Inport
  Bus Creator : BusCreator  Inputs=3
  Bus Selector1 : BusSelector  OutputSignals=Baro_Data.timestamp,Baro_Data.h_R_m
  Second Order LPF : FMT_Model_Lib/Filter/Second Order LPF  fc=5  zeta=0.707
      settings: SourceProductName=FMT Toolbox
  Signal Copy1 : SignalConversion  OverrideOpt=off
  Signal Copy3 : SignalConversion  OverrideOpt=off
  Baro_Meas : Outport  VectorParamsAs1DForOutWhenUnconnected=off
  wires:
  Sensor_Data/1 -> Bus Selector1/1
  Bus Selector1/2 -> Signal Copy1/1  "<h_R_m>"
  Bus Creator/1 -> Baro_Meas/1
  Bus Selector1/1 -> Signal Copy3/1  "<timestamp>"
  Signal Copy3/1 -> Bus Creator/1  "timestamp_ms"
  Signal Copy1/1 -> Second Order LPF/1, Bus Creator/2  "h_R_m"
  Second Order LPF/1 -> Bus Creator/3  "h_R_filter_m"

== system INS/Data_Fusion/Translation_Filter/TF_Data_PreProcess/Sensor_Process/TF_Sensor_Measures/GPS_Meas ==
  Sensor_Data : Inport
  Bus Creator : BusCreator  Inputs=12
  Bus Selector : BusSelector  OutputSignals=GPS_Data.dx_dlat,GPS_Data.dy_dlon,GPS_Data.dz_dh,GPS_Data.lat_rad,GPS_Data.lon_rad,GPS_Data.height_m,GPS_Data.vn_mPs,GPS_Data.ve_mPs,GPS_Data.vd_mPs,GPS_Data.timestamp_ms,GPS_Data.spd_quality,GPS_Data.pos_quality
  Signal Copy{,1..11} (12 alike) : SignalConversion  OverrideOpt=off
  GPS_Meas : Outport  VectorParamsAs1DForOutWhenUnconnected=off
  wires:
  Bus Selector/11 -> Signal Copy10/1  "<spd_quality>"
  Signal Copy9/1 -> Bus Creator/10  "timestamp_ms"
  Signal Copy8/1 -> Bus Creator/9  "vd_mPs"
  Signal Copy7/1 -> Bus Creator/8  "ve_mPs"
  Signal Copy6/1 -> Bus Creator/7  "vn_mPs"
  Signal Copy5/1 -> Bus Creator/6  "h_m"
  Signal Copy4/1 -> Bus Creator/5  "lon_rad"
  Signal Copy3/1 -> Bus Creator/4  "lat_rad"
  Signal Copy2/1 -> Bus Creator/3  "dz_dh"
  Signal Copy1/1 -> Bus Creator/2  "dy_dlon"
  Signal Copy/1 -> Bus Creator/1  "dx_dlat"
  Bus Selector/10 -> Signal Copy9/1  "<timestamp_ms>"
  Bus Selector/9 -> Signal Copy8/1  "<vd_mPs>"
  Bus Selector/8 -> Signal Copy7/1  "<ve_mPs>"
  Bus Selector/7 -> Signal Copy6/1  "<vn_mPs>"
  Bus Selector/6 -> Signal Copy5/1  "<height_m>"
  Bus Selector/5 -> Signal Copy4/1  "<lon_rad>"
  Bus Selector/4 -> Signal Copy3/1  "<lat_rad>"
  Bus Selector/3 -> Signal Copy2/1  "<dz_dh>"
  Bus Selector/2 -> Signal Copy1/1  "<dy_dlon>"
  Bus Selector/1 -> Signal Copy/1  "<dx_dlat>"
  Bus Creator/1 -> GPS_Meas/1
  Sensor_Data/1 -> Bus Selector/1
  Bus Selector/12 -> Signal Copy11/1  "<pos_quality>"
  Signal Copy10/1 -> Bus Creator/11  "spd_quality"
  Signal Copy11/1 -> Bus Creator/12  "pos_quality"

== system INS/Data_Fusion/Translation_Filter/TF_Data_PreProcess/Sensor_Process/TF_Sensor_Measures/OpticalFlow_Meas ==
  Sensor_Data : Inport
  Rotation_Data : Inport  Port=2
  Bus Creator : BusCreator  Inputs=3
  Bus Selector : BusSelector  OutputSignals=M_CO
  Bus Selector1 : BusSelector  OutputSignals=OpticalFlow_Data.timestamp
  Bus Selector2 : BusSelector  OutputSignals=OpticalFlow_Data.vx,OpticalFlow_Data.vy
  Constant : Constant  Value=0  OutDataTypeStr=single
  Multiply : Product  Multiplication=Matrix(*)
  Mux : Mux  Inputs=3
  Selector : Selector  InputPortWidth=3  IndexOptions=Index vector (dialog)  Indices=1  OutputSizes=1
  Selector1 : Selector  InputPortWidth=3  IndexOptions=Index vector (dialog)  Indices=2  OutputSizes=1
  Signal Copy3 : SignalConversion  OverrideOpt=off
  Transpose : Math  Operator=transpose  SignedPower=on  SaturateOnIntegerOverflow=on
  OptFlow_Meas : Outport  VectorParamsAs1DForOutWhenUnconnected=off
  wires:
  Sensor_Data/1 -> Bus Selector2/1, Bus Selector1/1
  Bus Creator/1 -> OptFlow_Meas/1
  Bus Selector1/1 -> Signal Copy3/1  "<timestamp>"
  Signal Copy3/1 -> Bus Creator/1  "timestamp_ms"
  Rotation_Data/1 -> Bus Selector/1
  Bus Selector/1 -> Transpose/1  "<M_CO>"
  Transpose/1 -> Multiply/1  "M_OC"
  Bus Selector2/1 -> Mux/1  "<vx>"
  Bus Selector2/2 -> Mux/2  "<vy>"
  Constant/1 -> Mux/3
  Mux/1 -> Multiply/2
  Selector/1 -> Bus Creator/2  "vx_O_mPs"
  Multiply/1 -> Selector1/1, Selector/1
  Selector1/1 -> Bus Creator/3  "vy_O_mPs"

== system INS/Data_Fusion/Translation_Filter/TF_Data_PreProcess/Sensor_Process/TF_Sensor_Measures/Rangefinder_Meas ==
  Sensor_Data : Inport
  Bus Creator : BusCreator  Inputs=2
  Bus Selector1 : BusSelector  OutputSignals=Rangefinder_Data.timestamp,Rangefinder_Data.distance
  Signal Copy1 : SignalConversion  OverrideOpt=off
  Signal Copy3 : SignalConversion  OverrideOpt=off
  Rf_Meas : Outport  VectorParamsAs1DForOutWhenUnconnected=off
  wires:
  Signal Copy1/1 -> Bus Creator/2  "h_AGL_m"
  Signal Copy3/1 -> Bus Creator/1  "timestamp_ms"
  Bus Selector1/1 -> Signal Copy3/1  "<timestamp>"
  Bus Creator/1 -> Rf_Meas/1
  Bus Selector1/2 -> Signal Copy1/1  "<distance>"
  Sensor_Data/1 -> Bus Selector1/1

== system INS/Data_Fusion/Translation_Filter/TF_Data_PreProcess/Sensor_Process/TF_Sensor_Status/Barometer_Status ==
  Sensor_Data : Inport
  Bus Creator : BusCreator  Inputs=1
  Bus Selector : BusSelector  OutputSignals=Baro_Data.baro_valid
  Signal Copy : SignalConversion  OverrideOpt=off
  Baro_Status : Outport  VectorParamsAs1DForOutWhenUnconnected=off
  wires:
  Bus Selector/1 -> Signal Copy/1  "<baro_valid>"
  Bus Creator/1 -> Baro_Status/1
  Sensor_Data/1 -> Bus Selector/1
  Signal Copy/1 -> Bus Creator/1  "baro_valid"

== system INS/Data_Fusion/Translation_Filter/TF_Data_PreProcess/Sensor_Process/TF_Sensor_Status/GPS_Status ==
  Sensor_Data : Inport
  Bus Creator : BusCreator  Inputs=4
  Bus Selector : BusSelector  OutputSignals=GPS_Data.GPS_valid,GPS_Data.spd_quality,GPS_Data.pos_quality,GPS_Data.alt_quality
  Relay : Relay  OnSwitchValue=0.7  OffSwitchValue=0.4
  Relay1 : Relay  OnSwitchValue=0.7  OffSwitchValue=0.6
  Relay2 : Relay  OnSwitchValue=0.7  OffSwitchValue=0.6
  Signal Copy : SignalConversion  OverrideOpt=off
  GPS_Status : Outport  VectorParamsAs1DForOutWhenUnconnected=off
  wires:
  Bus Creator/1 -> GPS_Status/1
  Relay1/1 -> Bus Creator/3  "pos_valid"
  Relay/1 -> Bus Creator/2  "spd_valid"
  Signal Copy/1 -> Bus Creator/1  "gps_vaid"
  Bus Selector/3 -> Relay1/1  "<pos_quality>"
  Bus Selector/2 -> Relay/1  "<spd_quality>"
  Bus Selector/1 -> Signal Copy/1  "<GPS_valid>"
  Sensor_Data/1 -> Bus Selector/1
  Bus Selector/4 -> Relay2/1  "<alt_quality>"
  Relay2/1 -> Bus Creator/4  "alt_valid"

== system INS/Data_Fusion/Translation_Filter/TF_Data_PreProcess/Sensor_Process/TF_Sensor_Status/OpticalFlow_Status ==
  Sensor_Data : Inport
  Bus Creator : BusCreator  Inputs=1
  Bus Selector : BusSelector  OutputSignals=OpticalFlow_Data.valid
  Signal Copy : SignalConversion  OverrideOpt=off
  OptFlow_Status : Outport  VectorParamsAs1DForOutWhenUnconnected=off
  wires:
  Signal Copy/1 -> Bus Creator/1  "optflow_valid"
  Sensor_Data/1 -> Bus Selector/1
  Bus Creator/1 -> OptFlow_Status/1
  Bus Selector/1 -> Signal Copy/1  "<valid>"

== system INS/Data_Fusion/Translation_Filter/TF_Data_PreProcess/Sensor_Process/TF_Sensor_Status/Rangefinder_Status ==
  Sensor_Data : Inport
  Bus Creator : BusCreator  Inputs=1
  Bus Selector : BusSelector  OutputSignals=Rangefinder_Data.valid
  Signal Copy : SignalConversion  OverrideOpt=off
  Rf_Status : Outport  VectorParamsAs1DForOutWhenUnconnected=off
  wires:
  Bus Selector/1 -> Signal Copy/1  "<valid>"
  Bus Creator/1 -> Rf_Status/1
  Sensor_Data/1 -> Bus Selector/1
  Signal Copy/1 -> Bus Creator/1  "rf_valid"

== system INS/Data_Fusion/Translation_Filter/TF_Data_PreProcess/Transfer_Filter_Control/Sensor_Valid/Horizon_Sensor_Valid ==
  Sensor_Enable : Inport
  Bus Selector1 : BusSelector  OutputSignals=horizon_select.gps_enable,horizon_select.optflow_enable
  Logical Operator : Logic  Operator=OR  AllPortsSameDT=off  OutDataTypeStr=boolean
  valid_hold : Subsystem  mask{time_out=1000}
      mask prompts: time_out "timeout in ms"
  valid_hold1 : Subsystem  mask{time_out=1000}
      mask prompts: time_out "timeout in ms"
  lon_lat_valid : Outport  VectorParamsAs1DForOutWhenUnconnected=off
  xy_R_valid : Outport  Port=2  VectorParamsAs1DForOutWhenUnconnected=off
  wires:
  Sensor_Enable/1 -> Bus Selector1/1
  Bus Selector1/1 -> Logical Operator/1, valid_hold/1(u)  "<gps_enable>"
  valid_hold/1(y) -> lon_lat_valid/1
  valid_hold1/1(y) -> xy_R_valid/1
  Bus Selector1/2 -> Logical Operator/2  "<optflow_enable>"
  Logical Operator/1 -> valid_hold1/1(u)

== system INS/Data_Fusion/Translation_Filter/TF_Data_PreProcess/Transfer_Filter_Control/Sensor_Valid/Vertical_Sensor_Valid ==
  Sensor_Enable : Inport
  Bus Selector1 : BusSelector  OutputSignals=vert_select.gps_enable,vert_select.baro_enable,vert_select.rf_enable
  Logical Operator : Logic  Operator=OR  Inputs=3  AllPortsSameDT=off  OutDataTypeStr=boolean
  valid_hold : Subsystem  mask{time_out=1000}
      mask prompts: time_out "timeout in ms"
  valid_hold1 : Subsystem  mask{time_out=1000}
      mask prompts: time_out "timeout in ms"
  valid_hold2 : Subsystem  mask{time_out=100}
      mask prompts: time_out "timeout in ms"
  altitude_valid : Outport  VectorParamsAs1DForOutWhenUnconnected=off
  h_R_valid : Outport  Port=2  VectorParamsAs1DForOutWhenUnconnected=off
  h_AGL_valid : Outport  Port=3  VectorParamsAs1DForOutWhenUnconnected=off
  wires:
  Sensor_Enable/1 -> Bus Selector1/1
  Bus Selector1/1 -> valid_hold/1(u), Logical Operator/1  "<gps_enable>"
  Bus Selector1/2 -> Logical Operator/2  "<baro_enable>"
  Logical Operator/1 -> valid_hold1/1(u)
  valid_hold/1(y) -> altitude_valid/1
  valid_hold1/1(y) -> h_R_valid/1
  Bus Selector1/3 -> Logical Operator/3, valid_hold2/1(u)  "<rf_enable>"
  valid_hold2/1(y) -> h_AGL_valid/1

== system INS/Data_Fusion/Translation_Filter/TF_Data_PreProcess/Transfer_Filter_Control/WGS84_Reference/Bus_Constructor ==
  WGS84_pos_ref : Inport
  WGS84_dpos_ref : Inport  Port=2
  WGS84_hgt_ref : Inport  Port=3
  WGS84_dhgt_ref : Inport  Port=4
  Bus Creator : BusCreator  Inputs=2
  Bus Creator1 : BusCreator  Inputs=3
  Bus Creator2 : BusCreator  Inputs=3
  Demux : Demux  Outputs=2
  Demux1 : Demux  Outputs=2
  WGS84_Ref : Outport  VectorParamsAs1DForOutWhenUnconnected=off
  wires:
  Bus Creator/1 -> WGS84_Ref/1
  Demux/1 -> Bus Creator1/1  "dx_dlat_0"
  Demux1/1 -> Bus Creator2/1  "lat_0_rad"
  Demux/2 -> Bus Creator1/2  "dy_dlon_0"
  Demux1/2 -> Bus Creator2/2  "lon_0_rad"
  Bus Creator2/1 -> Bus Creator/2  "WGS84_pos_ref"
  WGS84_dhgt_ref/1 -> Bus Creator1/3  "dz_dh_0"
  WGS84_hgt_ref/1 -> Bus Creator2/3  "h_0_m"
  Bus Creator1/1 -> Bus Creator/1  "WGS84_derivatives_ref"
  WGS84_dpos_ref/1 -> Demux/1
  WGS84_pos_ref/1 -> Demux1/1

== system INS/Data_Fusion/Translation_Filter/TF_Data_PreProcess/Transfer_Filter_Control/WGS84_Reference/Bus_Select ==
  Sensor_Meas : Inport
  Bus Selector1 : BusSelector  OutputSignals=GPS_Meas.dx_dlat,GPS_Meas.dy_dlon,GPS_Meas.dz_dh,GPS_Meas.lat_rad,GPS_Meas.lon_rad,GPS_Meas.h_m
  Mux : Mux  Inputs=3
  Mux1 : Mux  Inputs=3
  WGS84_derivatives : Outport  VectorParamsAs1DForOutWhenUnconnected=off
  WGS84_position : Outport  Port=2  VectorParamsAs1DForOutWhenUnconnected=off
  wires:
  Mux1/1 -> WGS84_position/1
  Sensor_Meas/1 -> Bus Selector1/1
  Mux/1 -> WGS84_derivatives/1
  Bus Selector1/6 -> Mux1/3  "<h_m>"
  Bus Selector1/5 -> Mux1/2  "<lon_rad>"
  Bus Selector1/4 -> Mux1/1  "<lat_rad>"
  Bus Selector1/3 -> Mux/3  "<dz_dh>"
  Bus Selector1/2 -> Mux/2  "<dy_dlon>"
  Bus Selector1/1 -> Mux/1  "<dx_dlat>"

== system INS/Data_Fusion/Translation_Filter/TF_Data_PreProcess/Transfer_Filter_Control/WGS84_Reference/Height_Ref ==
  Translation_Data : Inport
  Sensor_Valid : Inport  Port=2
  WGS84_derivatives : Inport  Port=3
  WGS84_position : Inport  Port=4
  Bus Selector1 : BusSelector  OutputSignals=h_R_m
  Bus Selector2 : BusSelector  OutputSignals=altitude_valid
  Delay : Delay  DelayLength=1
  Delay1 : Delay  DelayLength=1
  Detect Rise Positive3 : simulink/Logic and Bit Operations/Detect Rise Positive  vinit=0  OutDataTypeStr=boolean
  Selector : Selector  InputPortWidth=3  IndexOptions=Index vector (dialog)  Indices=3  OutputSizes=1
  Selector1 : Selector  InputPortWidth=3  IndexOptions=Index vector (dialog)  Indices=3  OutputSizes=1
  Sum : Sum  Inputs=|+-
  Switch1 : Switch  Criteria=u2 > Threshold
  Switch4 : Switch  Criteria=u2 > Threshold
  WGS84_hgt_ref : Outport  VectorParamsAs1DForOutWhenUnconnected=off
  WGS84_dhgt_ref : Outport  Port=2  VectorParamsAs1DForOutWhenUnconnected=off
  wires:
  Delay1/1 -> Switch4/3
  Switch4/1 -> WGS84_hgt_ref/1, Delay1/1
  Detect Rise Positive3/1 -> Switch1/2, Switch4/2
  Bus Selector2/1 -> Detect Rise Positive3/1  "<altitude_valid>"
  WGS84_derivatives/1 -> Selector/1
  Switch1/1 -> WGS84_dhgt_ref/1, Delay/1
  Delay/1 -> Switch1/3
  Sensor_Valid/1 -> Bus Selector2/1
  Translation_Data/1 -> Bus Selector1/1
  Sum/1 -> Switch4/1
  WGS84_position/1 -> Selector1/1
  Selector/1 -> Switch1/1
  Selector1/1 -> Sum/1
  Bus Selector1/1 -> Sum/2  "<h_R_m>"

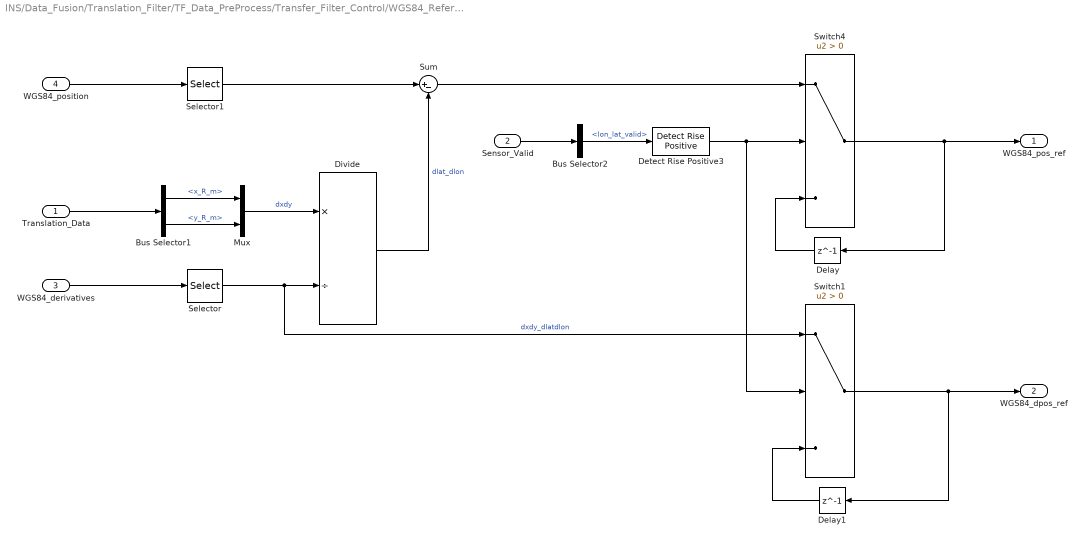
== system INS/Data_Fusion/Translation_Filter/TF_Data_PreProcess/Transfer_Filter_Control/WGS84_Reference/Position_Ref ==
  Translation_Data : Inport
  Sensor_Valid : Inport  Port=2
  WGS84_derivatives : Inport  Port=3
  WGS84_position : Inport  Port=4
  Bus Selector1 : BusSelector  OutputSignals=x_R_m,y_R_m
  Bus Selector2 : BusSelector  OutputSignals=lon_lat_valid
  Delay : Delay  DelayLength=1
  Delay1 : Delay  DelayLength=1
  Detect Rise Positive3 : simulink/Logic and Bit Operations/Detect Rise Positive  vinit=0  OutDataTypeStr=boolean
  Divide : Product  Inputs=*/
  Mux : Mux  Inputs=2
  Selector : Selector  InputPortWidth=3  IndexOptions=Index vector (dialog)  Indices=[1 2]  OutputSizes=1
  Selector1 : Selector  InputPortWidth=3  IndexOptions=Index vector (dialog)  Indices=[1 2]  OutputSizes=1
  Sum : Sum  Inputs=|+-
  Switch1 : Switch  Criteria=u2 > Threshold
  Switch4 : Switch  Criteria=u2 > Threshold
  WGS84_pos_ref : Outport  VectorParamsAs1DForOutWhenUnconnected=off
  WGS84_dpos_ref : Outport  Port=2  VectorParamsAs1DForOutWhenUnconnected=off
  wires:
  Delay/1 -> Switch4/3
  Bus Selector1/1 -> Mux/1  "<x_R_m>"
  Switch4/1 -> WGS84_pos_ref/1, Delay/1
  Mux/1 -> Divide/1  "dxdy"
  Detect Rise Positive3/1 -> Switch1/2, Switch4/2
  Bus Selector2/1 -> Detect Rise Positive3/1  "<lon_lat_valid>"
  WGS84_derivatives/1 -> Selector/1
  Switch1/1 -> Delay1/1, WGS84_dpos_ref/1
  Delay1/1 -> Switch1/3
  Sensor_Valid/1 -> Bus Selector2/1
  Translation_Data/1 -> Bus Selector1/1
  Sum/1 -> Switch4/1
  Bus Selector1/2 -> Mux/2  "<y_R_m>"
  Divide/1 -> Sum/2  "dlat_dlon"
  WGS84_position/1 -> Selector1/1
  Selector/1 -> Switch1/1, Divide/2  "dxdy_dlatdlon"
  Selector1/1 -> Sum/1

== system INS/Sensor_PreProcess/MAG_PreProcess/Mag_Data_Process/Mag_Quality_Estimate/Mag_Quality/Inclination_Quality_Estimate ==
  nominal_inc_deg : Inport
  mag_normalized_O : Inport  Port=2
  Abs1 : Abs
  Constant2 : Constant  OutDataTypeStr=Inherit: Inherit via back propagation
  Gain1 : Gain  Gain=pi/180
  Saturation : Saturate  UpperLimit=1  LowerLimit=0
  Selector : Selector  InputPortWidth=3  IndexOptions=Index vector (dialog)  Indices=[1 2]  OutputSizes=1
  Selector1 : Selector  InputPortWidth=3  IndexOptions=Index vector (dialog)  Indices=3  OutputSizes=1
  Subtract : Sum  Inputs=+-
  Sum3 : Sum  Inputs=+-|
  Trigonometric Function : Trigonometry  Operator=atan2
  Vector Modulus : FMT_Model_Lib/Math/Vector Modulus
      settings: SourceProductName=FMT Toolbox
  gain : Gain  Gain=2
  inclination_quality : Outport  VectorParamsAs1DForOutWhenUnconnected=off
  wires:
  mag_normalized_O/1 -> Selector1/1, Selector/1
  Trigonometric Function/1 -> Subtract/2
  Vector Modulus/1 -> Trigonometric Function/2
  Abs1/1 -> gain/1
  gain/1 -> Sum3/2
  Gain1/1 -> Subtract/1
  Subtract/1 -> Abs1/1
  Constant2/1 -> Sum3/1
  nominal_inc_deg/1 -> Gain1/1
  Sum3/1 -> Saturation/1
  Selector/1 -> Vector Modulus/1
  Selector1/1 -> Trigonometric Function/1
  Saturation/1 -> inclination_quality/1

== system INS/Sensor_PreProcess/MAG_PreProcess/Mag_Data_Process/Mag_Quality_Estimate/Mag_Quality/Intensity_Quality_Estimate ==
  mag_normalized_O : Inport
  Abs : Abs
  Constant1 : Constant  OutDataTypeStr=Inherit: Inherit via back propagation
  Nominal_Magnitude : Constant  OutDataTypeStr=Inherit: Inherit via back propagation
  Saturation : Saturate  UpperLimit=1  LowerLimit=0
  Subtract : Sum  Inputs=+-
  Sum : Sum  Inputs=+-|
  Vector Modulus : FMT_Model_Lib/Math/Vector Modulus
      settings: SourceProductName=FMT Toolbox
  gain : Gain
  intensity_quality : Outport  VectorParamsAs1DForOutWhenUnconnected=off
  wires:
  Constant1/1 -> Sum/1
  Vector Modulus/1 -> Subtract/2
  Subtract/1 -> Abs/1
  Sum/1 -> Saturation/1
  Nominal_Magnitude/1 -> Subtract/1
  Saturation/1 -> intensity_quality/1
  Abs/1 -> gain/1  "magnitude_error"
  gain/1 -> Sum/2
  mag_normalized_O/1 -> Vector Modulus/1

== system INS/Data_Fusion/Rotation_Filter/AHRS/Correct/Attitude_Correction/Attitude_Correct/Acc_Correct ==
  acc_meas_valid : Inport
  acc_meas_O_mPs2 : Inport  Port=2
  acc_est_O_mPs2 : Inport  Port=3
  Heading_Correct : Subsystem
  Sum : Sum  Inputs=|++
  Verticle_Correct : Subsystem
  att_correct : Outport  VectorParamsAs1DForOutWhenUnconnected=off
  wires:
  acc_meas_valid/1 -> Heading_Correct/3(acc_meas_valid)
  Verticle_Correct/1(vert_correct) -> Sum/1  "vert_correct"
  Heading_Correct/1(heading_correct) -> Sum/2  "heading_correct"
  acc_meas_O_mPs2/1 -> Verticle_Correct/2(acc_meas_O_mPs2), Heading_Correct/2(acc_meas_O_mPs2)
  acc_est_O_mPs2/1 -> Verticle_Correct/1(acc_est_O_mPs2), Heading_Correct/1(acc_est_O_mPs2)
  Sum/1 -> att_correct/1

== system INS/Data_Fusion/Rotation_Filter/AHRS/Correct/Attitude_Correction/Attitude_Correct/Acc_Estimator ==
  Sensor_Data : Inport
  Rotation_Data : Inport  Port=2
  Estimate_Acc : Subsystem
  Measure_Acc : Subsystem
  Multiply : Product  OutDataTypeStr=single
  Sum2 : Sum  Inputs=++|
  gravity : Constant  Value=[0;0;-INS_CONST.g]  VectorParams1D=off  OutDataTypeStr=single
  acc_meas_valid : Outport  VectorParamsAs1DForOutWhenUnconnected=off
  acc_meas_O_mPs2 : Outport  Port=2  VectorParamsAs1DForOutWhenUnconnected=off
  acc_est_O_mPs2 : Outport  Port=3  VectorParamsAs1DForOutWhenUnconnected=off
  wires:
  Measure_Acc/1(gps_meas_valid) -> Estimate_Acc/1(gps_meas_valid), acc_meas_valid/1, Multiply/1
  Sum2/1 -> acc_meas_O_mPs2/1
  Sensor_Data/1 -> Estimate_Acc/2(Sensor_Data), Measure_Acc/1(Sensor_Data)
  gravity/1 -> Sum2/1
  Multiply/1 -> Sum2/2
  Measure_Acc/2(gps_meas_acc) -> Multiply/2
  Rotation_Data/1 -> Estimate_Acc/3(Rotation_Data)
  Estimate_Acc/1(acc_est_O_mPs2) -> acc_est_O_mPs2/1

== system INS/Data_Fusion/Rotation_Filter/AHRS/Correct/Attitude_Correction/Mag_Correct/Subsystem ==
  M_OB : Inport
  mag_B : Inport  Port=2
  Rotation_Data : Inport  Port=3
  Add : Sum
  Atan2 : Trigonometry  Operator=atan2
  Bus Selector : BusSelector  OutputSignals=psi_rad
  Demux : Demux  Outputs=3
  Gain : Gain  Gain=-1
  MX Product1 : Product  Multiplication=Matrix(*)  RndMeth=Simplest
  Terminator : Terminator
  Terminator1 : Terminator
  wires:
  Demux/3 -> Terminator1/1
  Atan2/1 -> Add/1
  Demux/1 -> Atan2/2
  MX Product1/1 -> Demux/1  "my_O"
  Gain/1 -> Atan2/1
  Add/1 -> Terminator/1  "mag_heading"
  Rotation_Data/1 -> Bus Selector/1
  Bus Selector/1 -> Add/2  "<psi_rad>"
  Demux/2 -> Gain/1
  mag_B/1 -> MX Product1/2
  M_OB/1 -> MX Product1/1
